simulink model "ADRC_FULL_SFUCTION"  (R2022b)
settings: Solver=VariableStepAuto  StartTime=0.0  StopTime=10.0  RelTol=1e-3
settings Model: Creator=12854  LastModifiedBy=12854

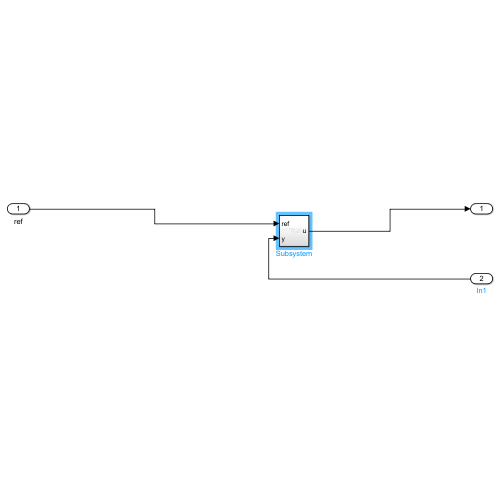
[thumbnail: Simulink's stored preview of the top-level diagram]
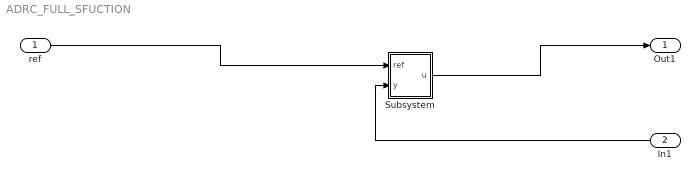
== system ADRC_FULL_SFUCTION ==
  ref : Inport
  In1 : Inport  Port=2
  Subsystem : Subsystem
  Out1 : Outport
  wires:
  ref/1 -> Subsystem/1(ref)
  In1/1 -> Subsystem/2(y)
  Subsystem/1(u) -> Out1/1

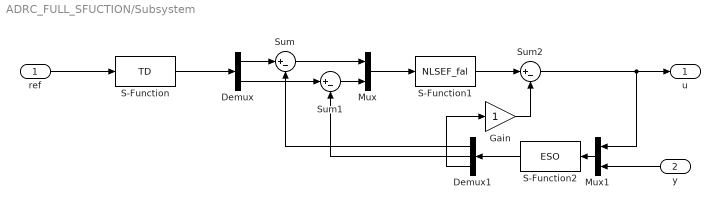
== system ADRC_FULL_SFUCTION/Subsystem ==
  ref : Inport
  y : Inport  Port=2
  Demux : Demux  Outputs=2
  Demux1 : Demux  Outputs=3
  Gain : Gain
  Mux : Mux  Inputs=2
  Mux1 : Mux  Inputs=2
  S-Function : S-Function  FunctionName=TD  Parameters=CtrlPara  SFunctionDeploymentMode=off  EnableBusSupport=off
  S-Function1 : S-Function  FunctionName=NLSEF_fal  Parameters=CtrlPara  SFunctionDeploymentMode=off  EnableBusSupport=off
  S-Function2 : S-Function  FunctionName=ESO  Parameters=CtrlPara  SFunctionDeploymentMode=off  EnableBusSupport=off
  Sum : Sum  Inputs=|+-
  Sum1 : Sum  Inputs=|+-
  Sum2 : Sum  Inputs=|+-
  u : Outport
  wires:
  S-Function1/1 -> Sum2/1
  Demux/1 -> Sum/1
  ref/1 -> S-Function/1
  S-Function/1 -> Demux/1
  Mux1/1 -> S-Function2/1
  S-Function2/1 -> Demux1/1
  Demux1/3 -> Gain/1
  Demux1/2 -> Sum1/2
  Gain/1 -> Sum2/2
  Sum/1 -> Mux/1
  Demux/2 -> Sum1/1
  Demux1/1 -> Sum/2
  Sum1/1 -> Mux/2
  Mux/1 -> S-Function1/1
  Sum2/1 -> u/1, Mux1/1
  y/1 -> Mux1/2
